simulink model "decline_h8000"  (R2023b)
settings: Solver=VariableStepAuto  StartTime=0.0  StopTime=30  RelTol=1e-3
undefined symbols (not defined in the file or in its folder): decline_h8000
settings Model: Creator=阿汪  LastModifiedBy=阿汪

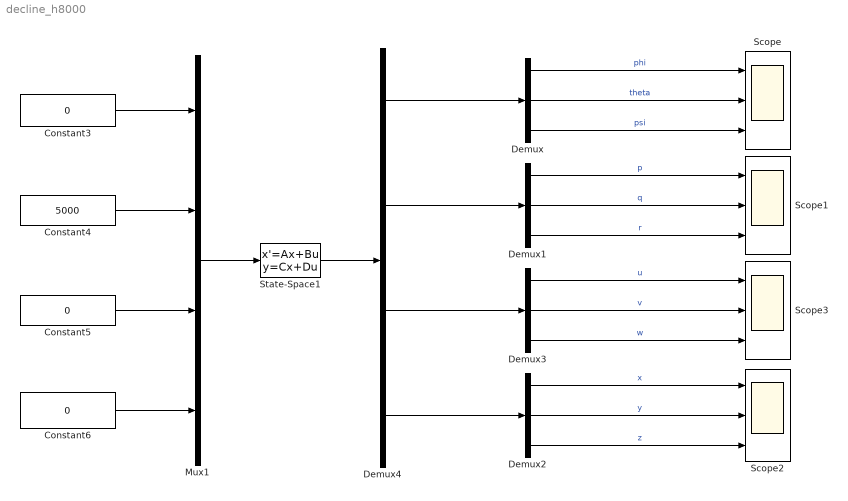
== system decline_h8000 ==
  Constant3 : Constant  Value=0
  Constant4 : Constant  Value=5000
  Constant5 : Constant  Value=0
  Constant6 : Constant  Value=0
  Demux{,1..3} (4 alike) : Demux  Outputs=3
  Demux4 : Demux
  Mux1 : Mux
  Scope{,1..3} (4 alike) : Scope  NumInputPorts=3
  State-Space1 : StateSpace  A=decline_h8000.A  B=decline_h8000.B  C=decline_h8000.C  D=decline_h8000.D  InitialCondition=[0;-0.05;0;0;0;0;200;0;0;0;0;-8000]
  wires:
  Demux2/2 -> Scope2/2  "y"
  Demux1/2 -> Scope1/2  "q"
  Mux1/1 -> State-Space1/1
  Demux3/1 -> Scope3/1  "u"
  Demux4/3 -> Demux3/1
  Demux/2 -> Scope/2  "theta"
  Constant5/1 -> Mux1/3
  Demux/1 -> Scope/1  "phi"
  Demux4/4 -> Demux2/1
  Demux/3 -> Scope/3  "psi"
  Demux4/1 -> Demux/1
  Demux1/1 -> Scope1/1  "p"
  Constant6/1 -> Mux1/4
  Constant4/1 -> Mux1/2
  Demux1/3 -> Scope1/3  "r"
  Constant3/1 -> Mux1/1
  State-Space1/1 -> Demux4/1
  Demux2/3 -> Scope2/3  "z"
  Demux3/2 -> Scope3/2  "v"
  Demux4/2 -> Demux1/1
  Demux3/3 -> Scope3/3  "w"
  Demux2/1 -> Scope2/1  "x"
